simulink model "Modell2"  (R2022b)
settings: Solver=VariableStepAuto  StartTime=0.0  StopTime=10.0  RelTol=1e-3
values from neighbouring files (symbols this model uses):
  K = 0.99    [Modell2_Params.m]
  T = 1    [Modell2_Params.m]
settings Model: Creator=bornk  LastModifiedBy=bornk

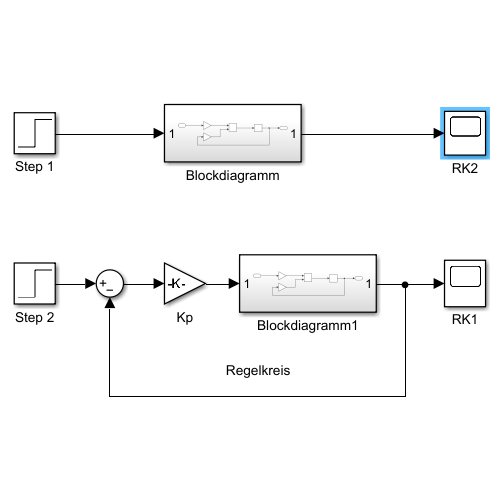
[thumbnail: Simulink's stored preview of the top-level diagram]
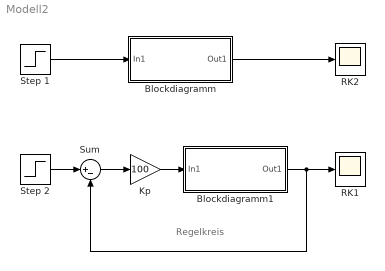
== system Modell2 ==
  note: Regelkreis
  Blockdiagramm : Subsystem
  Blockdiagramm1 : Subsystem
  Kp : Gain  Gain=100
  RK1 : Scope
  RK2 : Scope
  Step 1 : Step  SampleTime=0
  Step 2 : Step  SampleTime=0
  Sum : Sum  Inputs=|+-
  wires:
  Step 1/1 -> Blockdiagramm/1(In1)
  Blockdiagramm/1(Out1) -> RK2/1
  Blockdiagramm1/1(Out1) -> Sum/2, RK1/1
  Step 2/1 -> Sum/1
  Kp/1 -> Blockdiagramm1/1(In1)
  Sum/1 -> Kp/1

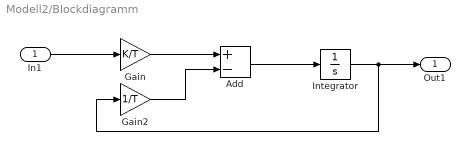
== system Modell2/Blockdiagramm ==
  In1 : Inport
  Add : Sum  Inputs=+-
  Gain : Gain  Gain=K/T
  Gain2 : Gain  Gain=1/T
  Integrator : Integrator
  Out1 : Outport
  wires:
  In1/1 -> Gain/1
  Gain/1 -> Add/1
  Gain2/1 -> Add/2
  Add/1 -> Integrator/1
  Integrator/1 -> Gain2/1, Out1/1

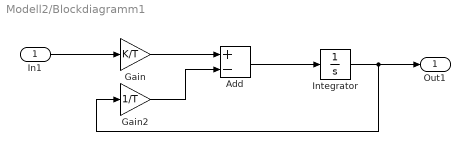
== system Modell2/Blockdiagramm1 ==
  In1 : Inport
  Add : Sum  Inputs=+-
  Gain : Gain  Gain=K/T
  Gain2 : Gain  Gain=1/T
  Integrator : Integrator
  Out1 : Outport
  wires:
  In1/1 -> Gain/1
  Gain/1 -> Add/1
  Gain2/1 -> Add/2
  Add/1 -> Integrator/1
  Integrator/1 -> Gain2/1, Out1/1
